simulink model "RefModel_Control"  (R2020a)
settings: Solver=ode1  StartTime=0.0  StopTime=1  FixedStep=dt  MaxStep=Ts  RelTol=1e-3
(part 1 of 3)
settings Model: Creator=sl  LastModifiedBy=a4327
settings DataIOCC: SaveOutput=off  SaveTime=off
settings OptimizationCC: DefaultParameterBehavior=Inlined  EnhancedBackFolding=on  PassReuseOutputArgsAs=Individual arguments  ZeroExternalMemoryAtStartup=off  ZeroInternalMemoryAtStartup=off  OptimizeBlockOrder=speed  DifferentSizesBufferReuse=on  OptimizationCustomize=off  EfficientTunableParamExpr=on
settings DebuggingCC: InheritedTsInSrcMsg=none  ParameterPrecisionLossMsg=none  ParameterTunabilityLossMsg=error  UnconnectedInputMsg=none  UnconnectedOutputMsg=none  UnconnectedLineMsg=none
settings HardwareCC: ProdBitPerPointer=32  ProdBitPerSizeT=32  ProdBitPerPtrDiffT=32  ProdLargestAtomicInteger=Long  ProdLargestAtomicFloat=Double  ProdWordSize=32  ProdHWDeviceType=ARM Compatible->ARM Cortex
settings ModelReferenceCC: ParallelModelReferenceMATLABWorkerInit=Copy Base Workspace  ModelReferenceNumInstancesAllowed=Single
settings SFSimCC: MATLABDynamicMemAlloc=off
settings RTWCC: SystemTargetFile=ert.tlc  GenCodeOnly=on  PackageGeneratedCodeAndArtifacts=on  TemplateMakefile=ert_default_tmf  GenerateReport=on  IncludeHyperlinkInReport=on  LaunchReport=on  GenerateTraceInfo=on  GenerateTraceReport=on  GenerateTraceReportSl=on  GenerateTraceReportSf=on  GenerateTraceReportEml=on
settings CodeAppCC: ForceParamTrailComments=on  IgnoreCustomStorageClasses=off  MaxIdLength=48  OperatorAnnotations=on  SimulinkDataObjDesc=on  SFDataObjDesc=on  MATLABFcnDesc=on  InsertBlockDesc=on  MATLABSourceComments=on
settings ERTTargetCC: TargetLangStandard=C99 (ISO)  GenerateSampleERTMain=on  LogVarNameModifier=none  SupportVariableSizeSignals=on  InlinedParameterPlacement=NonHierarchical  ERTCustomFileTemplate=example_file_process.tlc  ERTFilePackagingFormat=Compact

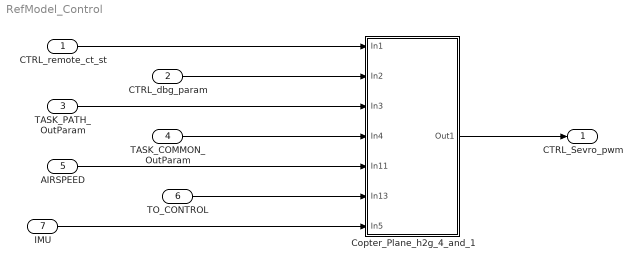
== system RefModel_Control ==
  CTRL_remote_ct_st : Inport  OutDataTypeStr=Bus: BUS_CTRL_remote_ct_st  BusOutputAsStruct=on
  CTRL_dbg_param : Inport  Port=2  OutDataTypeStr=Bus: BUS_CTRL_dbg_param  BusOutputAsStruct=on
  TASK_PATH_OutParam : Inport  Port=3  OutDataTypeStr=Bus: BUS_TASK_PATH_OutParam  BusOutputAsStruct=on
  TASK_COMMON_OutParam : Inport  Port=4  OutDataTypeStr=Bus: BUS_TASK_COMMON_OutParam  BusOutputAsStruct=on
  AIRSPEED : Inport  Port=5  OutDataTypeStr=Bus: BUS_AIRSPEED  BusOutputAsStruct=on
  TO_CONTROL : Inport  Port=6  OutDataTypeStr=Bus: BUS_TO_CONTROL  BusOutputAsStruct=on
  IMU : Inport  Port=7  OutDataTypeStr=Bus: BUS_IMU  BusOutputAsStruct=on
  Copter_Plane_h2g_4_and_1 : Subsystem
  CTRL_Sevro_pwm : Outport  OutDataTypeStr=Bus: BUS_CTRL_Sevro_pwm
  wires:
  TO_CONTROL/1 -> Copter_Plane_h2g_4_and_1/6(In13)
  TASK_PATH_OutParam/1 -> Copter_Plane_h2g_4_and_1/3(In3)
  Copter_Plane_h2g_4_and_1/1(Out1) -> CTRL_Sevro_pwm/1
  AIRSPEED/1 -> Copter_Plane_h2g_4_and_1/5(In11)
  IMU/1 -> Copter_Plane_h2g_4_and_1/7(In5)
  TASK_COMMON_OutParam/1 -> Copter_Plane_h2g_4_and_1/4(In4)
  CTRL_remote_ct_st/1 -> Copter_Plane_h2g_4_and_1/1(In1)
  CTRL_dbg_param/1 -> Copter_Plane_h2g_4_and_1/2(In2)
